simulink model "full_model"  (R2021a)
settings: Solver=FixedStepAuto  StartTime=0.0  StopTime=conf.cycle.stop  FixedStep=conf.time.step  RelTol=1e-3
InitFcn:
  | full_model_init
values from neighbouring files (symbols this model uses):
  bottomCool = abs(conf.cooling.b.x) + abs(conf.cooling.b.y) == 1    [full_model_init.m]
  cellsP = conf.cells.p    [full_model_init.m]
  cellsS = conf.modules.x*conf.modules.y*conf.cells.s    [full_model_init.m]
  elecC1 = C1_matrix*elecCellCap/cellCapGiant    [full_model_init.m]
  elecCellCap = 60    [full_model_init.m]
  elecInitSOC = (1 - variation)*socAve + 2*variation*socAve*rand(cellsS,cellsP)    [full_model_init.m]
  elecLoadDenomInds = 0    [full_model_init.m]
  elecLoadTerm12Inds = 0    [full_model_init.m]
  elecLoadTerm1Inds = 0    [full_model_init.m]
  elecLoadTerm2Inds = 0    [full_model_init.m]
  elecLoadTerm3Inds = 0    [full_model_init.m]
  elecOCV = Em_matrix    [full_model_init.m]
  elecR0 = R1_matrix*cellCapGiant/elecCellCap    [full_model_init.m]
  elecR1 = R2_matrix*cellCapGiant/elecCellCap    [full_model_init.m]
  elecSOCBreak = SOC_breakpoints    [full_model_init.m]
  elecTempBreak = Temp_breakpoints    [full_model_init.m]
  maxFlow = min([maxFlowX maxFlowY])    [full_model_init.m]
  mdotDistX = mdotDistX*flowMult    [full_model_init.m]
  mdotDistY = mdotDistY*flowMult    [full_model_init.m]
  n = n + 1    (= 5)    [plot_lines.m]    (also in plot_volumes.m = 2)
  tempAmb = conf.bound.amb    [full_model_init.m]    (also in order_reduction_script.m = data.tempAmb)
  tempTarget = 25    [full_model_init.m]
  thermBoundXA = conf.bound.amb    [full_model_init.m]
  thermBoundXB = conf.bound.amb    [full_model_init.m]
  thermBoundYA = conf.bound.amb    [full_model_init.m]
  thermBoundYB = conf.bound.amb    [full_model_init.m]
  thermBoundZA = conf.bound.amb    [full_model_init.m]
  thermBoundZB = conf.bound.amb    [full_model_init.m]
  thermCellVols = (thermHeatInds ~= 0)    [full_model_init.m]
  thermCp = matDict.Mass_Cp(thermMatID)    [full_model_init.m]
  thermHeatCellToVol = 1/(conf.regions.l*conf.regions.w*conf.regions.t)    [full_model_init.m]
  thermInitTemp = tempAmb*ones(thermDims)+ conf.bound.initBias    [full_model_init.m]
  thermKx = tempK.x    [full_model_init.m]
  thermKy = tempK.y    [full_model_init.m]
  thermKz = tempK.z    [full_model_init.m]
  thermM = rho.*V    [full_model_init.m]
  thermTempInds = zeros(conf.regions.l*conf.regions.w*conf.regions.t,1,cellsS*cellsP)    [full_model_init.m]
  topCool = abs(conf.cooling.t.x) + abs(conf.cooling.t.y) == 1    [full_model_init.m]
  vehAf = 3.15    [full_model_init.m]
  vehCd = 0.28    [full_model_init.m]
  vehM = 2565    [full_model_init.m]
  vehPowerMult = modelEnergy/packEnergy    [full_model_init.m]
undefined symbols (not defined in the file or in its folder): conf, radAirVelBreakPoints, radCoolFlowBreakPoints, radNomFlowMatrix, refAirVelBreakPoints, refCoolFlowBreakPoints, refCoolInTempBreakPoints, refTempOutMatrix, thermDims
libraries: visionstatistics x1
settings Model: Creator=sjtho  LastModifiedBy=sjtho
settings OptimizationCC: OptimizeBlockIOStorage=off  OptimizeDataStoreBuffers=off  BusAssignmentInplaceUpdate=off
settings DebuggingCC: UniqueDataStoreMsg=error  SFUnexpectedBacktrackingDiag=warning  SFNoUnconditionalDefaultTransitionDiag=warning
settings RTWCC: GenerateReport=on  BuildConfiguration=Debug  LaunchReport=on
settings CodeAppCC: ForceParamTrailComments=on  MATLABSourceComments=on  EnableCustomComments=on
settings GRTTargetCC: CombineSignalStateStructs=on  SupportVariableSizeSignals=on  MultiInstanceErrorCode=Warning

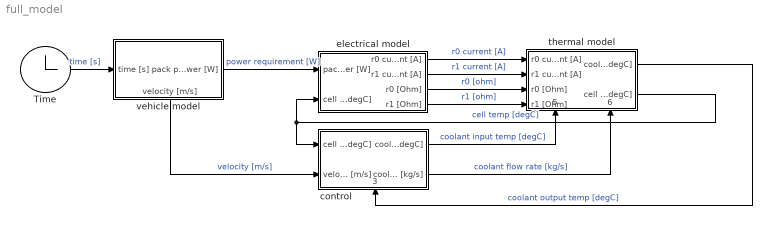
== system full_model ==
  Time : Clock
  control : Subsystem
      settings: PortSchema="{\"entries\":[{\"content\":{\"sides\":[{\"content\":{\"connectorIds\":[\"In1\",\"In2\"]},\"type\":\"ConnectorPlacement.EquallySpacedRectSide\",\"uuid\":\"22f80eaa-bb46-4281-9ec1-3970c1bac2a3\"},{\"content\":{\"connectorIds\":[\"Out1\",\"Out2\"],\"side\":\"RIGHT\"},\"type\":\"ConnectorPlacement.EquallySpacedRectSide\",\"uuid\":\"e76f71c5-d41f-442d-b655-b3bc32395443\"},{\"content\":{\"connectorIds\":[],\"side\":\"TOP\"},\"type\":\"ConnectorPlacement.EquallySpacedRectSide\",\"uuid\":\"e3a9d903-5780-49ee-b4b3-f001d4a3722b\"},{\"content\":{\"connectorIds\":[\"In3\"],\"side\":\"BOTTOM\"},\"type\":\"ConnectorPlacement.EquallySpacedRectSide\",\"uuid\":\"8a36595f-00ae-4362-a59c-271e32328d9e\"}]},\"type\":\"ConnectorPlacement.EquallySpacedConnector\",\"uuid\":\"d37af0d9-ec54-4f0d-b375-47d72f1b804c\"}],\"packageUris\":[\"http://schema.mathworks.com/mf0/Connector/R2020b\"],\"version\":\"1.0\"}"
      mask Display: disp(['Control and ' newline 'Thermal management'])
  electrical model : Subsystem
      mask Display: disp('Electrical Model')
  thermal model : Subsystem
      settings: PortSchema="{\"entries\":[{\"content\":{\"sides\":[{\"content\":{\"connectorIds\":[\"In1\",\"In2\",\"In3\",\"In4\"]},\"type\":\"ConnectorPlacement.EquallySpacedRectSide\",\"uuid\":\"85abd361-fdf9-4e50-9692-c6cfc682c3ac\"},{\"content\":{\"connectorIds\":[\"Out1\",\"Out2\"],\"side\":\"RIGHT\"},\"type\":\"ConnectorPlacement.EquallySpacedRectSide\",\"uuid\":\"50be5dc9-6285-4d3d-a0f1-610cf70c20d6\"},{\"content\":{\"connectorIds\":[],\"side\":\"TOP\"},\"type\":\"ConnectorPlacement.EquallySpacedRectSide\",\"uuid\":\"1bb98c42-8893-43bf-953b-d262aeaa61fe\"},{\"content\":{\"connectorIds\":[\"In5\",\"In6\"],\"side\":\"BOTTOM\"},\"type\":\"ConnectorPlacement.EquallySpacedRectSide\",\"uuid\":\"83d18484-4c30-41fd-9096-006931d5d21f\"}]},\"type\":\"ConnectorPlacement.EquallySpacedConnector\",\"uuid\":\"8afb65a4-2410-4c66-9cd3-3c36ab441c83\"}],\"packageUris\":[\"http://schema.mathworks.com/mf0/Connector/R2020b\"],\"version\":\"1.0\"}"
      mask Display: disp('Thermal Model')
  vehicle model : Subsystem
      settings: PortSchema="{\"entries\":[{\"content\":{\"sides\":[{\"content\":{\"connectorIds\":[\"In1\"]},\"type\":\"ConnectorPlacement.EquallySpacedRectSide\",\"uuid\":\"cf313784-55fc-4068-b83a-27fead484f77\"},{\"content\":{\"connectorIds\":[\"Out1\"],\"side\":\"RIGHT\"},\"type\":\"ConnectorPlacement.EquallySpacedRectSide\",\"uuid\":\"2b8b7e96-e7dc-4089-926d-80148fade29f\"},{\"content\":{\"connectorIds\":[],\"side\":\"TOP\"},\"type\":\"ConnectorPlacement.EquallySpacedRectSide\",\"uuid\":\"332287a3-327f-4bf8-9290-89809e483fea\"},{\"content\":{\"connectorIds\":[\"Out2\"],\"side\":\"BOTTOM\"},\"type\":\"ConnectorPlacement.EquallySpacedRectSide\",\"uuid\":\"f07f6670-fe7e-40c0-9cd8-41a00d5f5993\"}]},\"type\":\"ConnectorPlacement.EquallySpacedConnector\",\"uuid\":\"6bd39f86-8f76-4883-86c4-8a861857bd9f\"}],\"packageUris\":[\"http://schema.mathworks.com/mf0/Connector/R2020b\"],\"version\":\"1.0\"}"
      mask Display: disp('Vehicle Model')
  wires:
  Time/1 -> vehicle model/1(time [s])  "time [s]"
  vehicle model/1(pack power [W]) -> electrical model/1(pack power [W])  "power requirement [W]"
  control/1(coolant input temp [degC]) -> thermal model/5(coolant input temp [degC])  "coolant input temp [degC]"
  control/2(coolant flow rate [kg/s]) -> thermal model/6(coolant flow rate [kg/s])  "coolant flow rate [kg/s]"
  thermal model/1(coolant output temp [degC]) -> control/3(coolant output temp [degC])  "coolant output temp [degC]"
  electrical model/1(r0 current [A]) -> thermal model/1(r0 current [A])  "r0 current [A]"
  electrical model/2(r1 current [A]) -> thermal model/2(r1 current [A])  "r1 current [A]"
  electrical model/3(r0 [Ohm]) -> thermal model/3(r0 [Ohm])  "r0 [ohm]"
  electrical model/4(r1 [Ohm]) -> thermal model/4(r1 [Ohm])  "r1 [ohm]"
  thermal model/2(cell temp [degC]) -> control/1(cell temp [degC]), electrical model/2(cell temp [degC])  "cell temp [degC]"
  vehicle model/2(velocity [m/s]) -> control/2(velocity [m/s])  "velocity [m/s]"

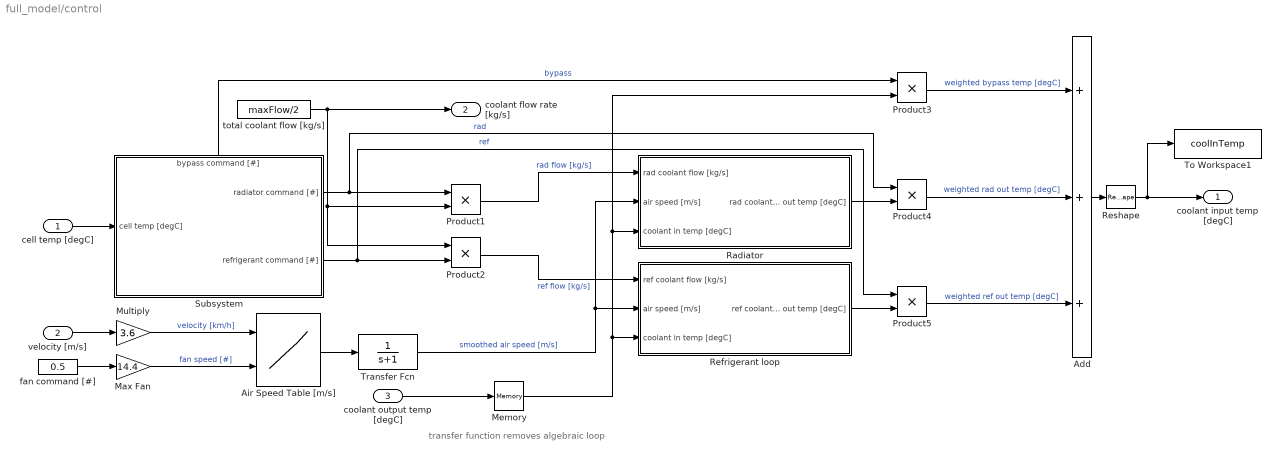
== system full_model/control ==
  note: transfer function removes algebraic loop
  cell temp [degC] : Inport
  velocity [m/s] : Inport  Port=2
  coolant output temp [degC] : Inport  Port=3
  Add : Sum  Inputs=+++
  Air Speed Table [m/s] : Lookup_n-D  BreakpointsForDimension1=[0 40 90 110 150 180 198]  BreakpointsForDimension2=[0 14.4]  IndexSearchMethod=Linear search  BeginIndexSearchUsingPreviousIndexResult=on  Table=[0 0.8 2.2 2.7 3.6 4.1 4.6; 1.5 2.3 3.2 3.5 4.3 4.8 5.1]'  InternalRulePriority=Speed  RndMeth=Simplest  InputSameDT=on
      settings: InputPortMap=u0,u1
  Max Fan : Gain  Gain=14.4
  Memory : Memory  InitialCondition=tempAmb + conf.bound.initBias
  Multiply : Gain  Gain=3.6
  Product{1..5} (5 alike) : Product
  Radiator : Subsystem
  Refrigerant loop : Subsystem
  Reshape : Reshape  OutputDimensionality=Customize  OutputDimensions=1
  Subsystem : Subsystem
      settings: PortSchema="{\"entries\":[{\"content\":{\"sides\":[{\"content\":{\"connectorIds\":[\"In1\"]},\"type\":\"ConnectorPlacement.EquallySpacedRectSide\",\"uuid\":\"39caf9d2-37e9-4ddb-8f89-28cdec2ac0f1\"},{\"content\":{\"connectorIds\":[\"Out1\",\"Out2\"],\"side\":\"RIGHT\"},\"type\":\"ConnectorPlacement.EquallySpacedRectSide\",\"uuid\":\"3cbc02da-b039-4e1d-b42e-efc08ec78021\"},{\"content\":{\"connectorIds\":[\"Out3\"],\"side\":\"TOP\"},\"type\":\"ConnectorPlacement.EquallySpacedRectSide\",\"uuid\":\"b4b3f97e-dd64-49e3-8c52-9947fb1a0732\"}]},\"type\":\"ConnectorPlacement.EquallySpacedConnector\",\"uuid\":\"4860c07b-2c7d-4cd4-976e-5c2ba4e5db64\"}],\"packageUris\":[\"http://schema.mathworks.com/mf0/Connector/R2020b\"],\"version\":\"1.0\"}"
  To Workspace1 : ToWorkspace  VariableName=coolInTemp  SaveFormat=Timeseries  SampleTime=conf.time.sample
  Transfer Fcn : TransferFcn  Denominator=[1 1]
  fan command [#] : Constant  Value=0.5
  total coolant flow [kg/s] : Constant  Value=maxFlow/2
  coolant input temp [degC] : Outport
  coolant flow rate [kg/s] : Outport  Port=2
  wires:
  Max Fan/1 -> Air Speed Table [m/s]/2  "fan speed [#]"
  velocity [m/s]/1 -> Multiply/1
  fan command [#]/1 -> Max Fan/1
  Multiply/1 -> Air Speed Table [m/s]/1  "velocity [km/h]"
  Air Speed Table [m/s]/1 -> Transfer Fcn/1
  cell temp [degC]/1 -> Subsystem/1(cell temp [degC])
  Subsystem/1(radiator command [#]) -> Product1/1, Product4/1  "rad"
  Subsystem/2(refrigerant command [#]) -> Product5/1, Product2/2  "ref"
  Product1/1 -> Radiator/1(rad coolant flow [kg/s])  "rad flow [kg/s]"
  Product2/1 -> Refrigerant loop/1(ref coolant flow [kg/s])  "ref flow [kg/s]"
  Transfer Fcn/1 -> Radiator/2(air speed [m/s]), Refrigerant loop/2(air speed [m/s])  "smoothed air speed [m/s]"
  coolant output temp [degC]/1 -> Memory/1
  Refrigerant loop/1(ref coolant out temp [degC]) -> Product5/2
  Radiator/1(rad coolant out temp [degC]) -> Product4/2
  Product4/1 -> Add/2  "weighted rad out temp [degC]"
  Product5/1 -> Add/3  "weighted ref out temp [degC]"
  Product3/1 -> Add/1  "weighted bypass temp [degC]"
  Subsystem/3(bypass command [#]) -> Product3/1  "bypass"
  total coolant flow [kg/s]/1 -> Product2/1, Product1/2, coolant flow rate [kg/s]/1
  Memory/1 -> Product3/2, Radiator/3(coolant in temp [degC]), Refrigerant loop/3(coolant in temp [degC])
  Add/1 -> Reshape/1
  Reshape/1 -> To Workspace1/1, coolant input temp [degC]/1

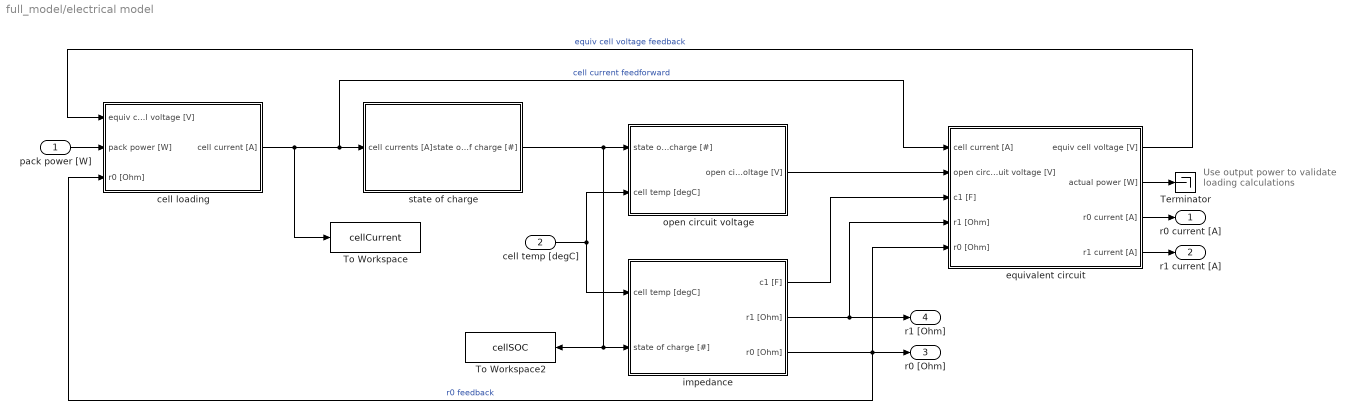
== system full_model/electrical model ==
  note: Use output power to validate loading calculations
  pack power [W] : Inport
  cell temp [degC] : Inport  Port=2
  Terminator : Terminator
  To Workspace : ToWorkspace  VariableName=cellCurrent  SaveFormat=Timeseries  SampleTime=conf.time.sample
  To Workspace2 : ToWorkspace  VariableName=cellSOC  SaveFormat=Timeseries  SampleTime=conf.time.sample
  cell loading : Subsystem
  equivalent circuit : Subsystem
  impedance : Subsystem
  open circuit voltage : Subsystem
  state of charge : Subsystem
  r0 current [A] : Outport
  r1 current [A] : Outport  Port=2
  r0 [Ohm] : Outport  Port=3
  r1 [Ohm] : Outport  Port=4
  wires:
  cell loading/1(cell current [A]) -> To Workspace/1, state of charge/1(cell currents [A]), equivalent circuit/1(cell current [A])  "cell current feedforward"
  cell temp [degC]/1 -> open circuit voltage/2(cell temp [degC]), impedance/1(cell temp [degC])
  state of charge/1(state of charge [#]) -> open circuit voltage/1(state of charge [#]), To Workspace2/1, impedance/2(state of charge [#])
  open circuit voltage/1(open circuit voltage [V]) -> equivalent circuit/2(open circuit voltage [V])
  equivalent circuit/2(actual power [W]) -> Terminator/1
  equivalent circuit/3(r0 current [A]) -> r0 current [A]/1
  equivalent circuit/4(r1 current [A]) -> r1 current [A]/1
  equivalent circuit/1(equiv cell voltage [V]) -> cell loading/1(equiv cell voltage [V])  "equiv cell voltage feedback"
  pack power [W]/1 -> cell loading/2(pack power [W])
  impedance/1(c1 [F]) -> equivalent circuit/3(c1 [F])
  impedance/2(r1 [Ohm]) -> r1 [Ohm]/1, equivalent circuit/4(r1 [Ohm])
  impedance/3(r0 [Ohm]) -> r0 [Ohm]/1, cell loading/3(r0 [Ohm]), equivalent circuit/5(r0 [Ohm])  "r0 feedback"

== system full_model/thermal model ==
  r0 current [A] : Inport
  r1 current [A] : Inport  Port=2
  r0 [Ohm] : Inport  Port=3
  r1 [Ohm] : Inport  Port=4
  coolant input temp [degC] : Inport  Port=5
  coolant flow rate [kg/s] : Inport  Port=6
  Sum1 : Sum  Inputs=|++
  cell temp : Subsystem
      mask Display: disp('Cell Temp')
  coolant flux : Subsystem
      mask Display: disp('Coolant Transfer')
  heat generation : Subsystem
      mask Display: disp('Heat Generation')
  coolant output temp [degC] : Outport
  cell temp [degC] : Outport  Port=2
  wires:
  cell temp/2(volume temp [degC]) -> coolant flux/3(volume temp [K])  "volume temp [degC]"
  coolant input temp [degC]/1 -> coolant flux/1(coolant input temp [K])
  coolant flow rate [kg/s]/1 -> coolant flux/2(coolant flow rate [kg/s])
  r0 current [A]/1 -> heat generation/1(r0 current [A])
  r1 current [A]/1 -> heat generation/2(r1 current [A])
  r0 [Ohm]/1 -> heat generation/3(r0 [Ohm])
  r1 [Ohm]/1 -> heat generation/4(r1 [Ohm])
  heat generation/1(volume heat generation [W]) -> Sum1/1  "volume heat generation [W]"
  cell temp/1(cell temp [degC]) -> cell temp [degC]/1
  Sum1/1 -> cell temp/1(net heat gain [W])  "net heat gain [W]"
  coolant flux/2(coolant output temp [degC]) -> coolant output temp [degC]/1
  coolant flux/1(volume coolant flux [W]) -> Sum1/2

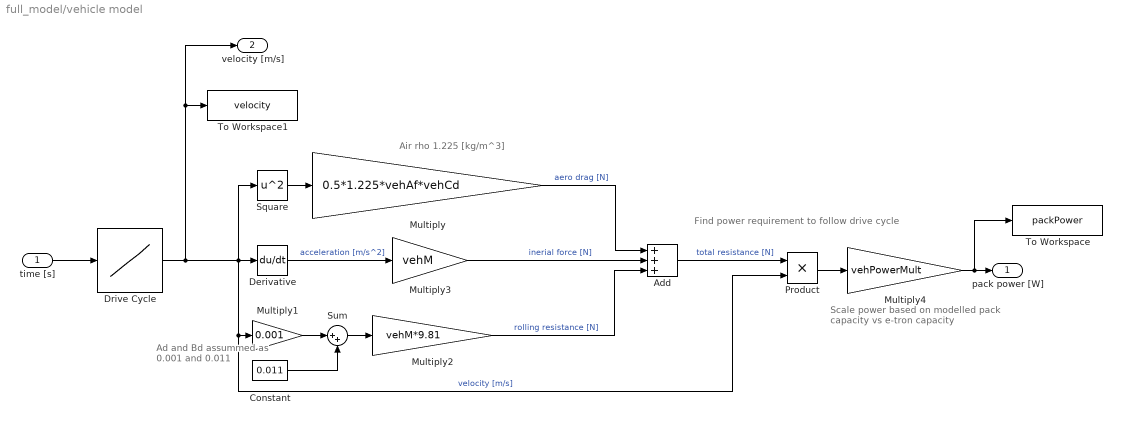
== system full_model/vehicle model ==
  note: Scale power based on modelled pack capacity vs e-tron capacity
  note: Ad and Bd assummed as 0.001 and 0.011
  note: Air rho 1.225 [kg/m^3]
  note: Find power requirement to follow drive cycle
  time [s] : Inport
  Add : Sum  Inputs=+++
  Constant : Constant  Value=0.011
  Derivative : Derivative
  Drive Cycle : Lookup_n-D  NumberOfTableDimensions=1  BreakpointsForDimension1=conf.cycle.time  Table=conf.cycle.vel  InterpMethod=Cubic spline  InternalRulePriority=Speed  RndMeth=Simplest  InputSameDT=on
  Multiply : Gain  Gain=0.5*1.225*vehAf*vehCd
  Multiply1 : Gain  Gain=0.001
  Multiply2 : Gain  Gain=vehM*9.81
  Multiply3 : Gain  Gain=vehM
  Multiply4 : Gain  Gain=vehPowerMult
  Product : Product
  Square : Math  Operator=square  SaturateOnIntegerOverflow=on
  Sum : Sum  Inputs=|++
  To Workspace : ToWorkspace  VariableName=packPower  SaveFormat=Timeseries  SampleTime=conf.time.sample
  To Workspace1 : ToWorkspace  VariableName=velocity  SaveFormat=Timeseries  SampleTime=conf.time.sample
  pack power [W] : Outport
  velocity [m/s] : Outport  Port=2
  wires:
  time [s]/1 -> Drive Cycle/1
  Multiply/1 -> Add/1  "aero drag [N]"
  Drive Cycle/1 -> velocity [m/s]/1, To Workspace1/1, Derivative/1, Multiply1/1, Product/2, Square/1  "velocity [m/s]"
  Add/1 -> Product/1  "total resistance [N]"
  Multiply3/1 -> Add/2  "inerial force [N]"
  Square/1 -> Multiply/1
  Multiply1/1 -> Sum/1
  Derivative/1 -> Multiply3/1  "acceleration [m/s^2]"
  Sum/1 -> Multiply2/1
  Constant/1 -> Sum/2
  Multiply2/1 -> Add/3  "rolling resistance [N]"
  Product/1 -> Multiply4/1
  Multiply4/1 -> To Workspace/1, pack power [W]/1

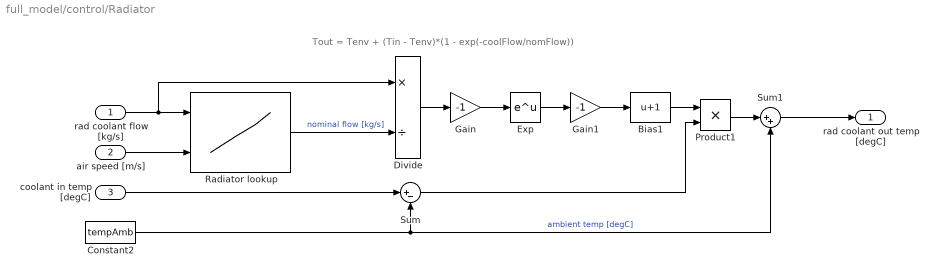
== system full_model/control/Radiator ==
  note: Tout = Tenv + (Tin - Tenv)*(1 - exp(-coolFlow/nomFlow))
  rad coolant flow [kg/s] : Inport
  air speed [m/s] : Inport  Port=2
  coolant in temp [degC] : Inport  Port=3
  Bias1 : Bias  Bias=1
  Constant2 : Constant  Value=tempAmb
  Divide : Product  Inputs=*/
  Exp : Math  SaturateOnIntegerOverflow=on
  Gain : Gain  Gain=-1
  Gain1 : Gain  Gain=-1
  Product1 : Product
  Radiator lookup : Lookup_n-D  BreakpointsForDimension1=radCoolFlowBreakPoints  BreakpointsForDimension2=radAirVelBreakPoints  BreakpointsForDimension3=refCoolInTempBreakPoints  Table=radNomFlowMatrix  InternalRulePriority=Speed  RndMeth=Simplest  InputSameDT=on
      settings: InputPortMap=u0,u1
  Sum : Sum  Inputs=|+-
  Sum1 : Sum  Inputs=|++
  rad coolant out temp [degC] : Outport
  wires:
  Radiator lookup/1 -> Divide/2  "nominal flow [kg/s]"
  Product1/1 -> Sum1/1
  rad coolant flow [kg/s]/1 -> Divide/1, Radiator lookup/1
  air speed [m/s]/1 -> Radiator lookup/2
  Divide/1 -> Gain/1
  Gain/1 -> Exp/1
  Exp/1 -> Gain1/1
  Gain1/1 -> Bias1/1
  Bias1/1 -> Product1/1
  coolant in temp [degC]/1 -> Sum/1
  Constant2/1 -> Sum1/2, Sum/2  "ambient temp [degC]"
  Sum/1 -> Product1/2
  Sum1/1 -> rad coolant out temp [degC]/1

== system full_model/control/Refrigerant loop ==
  ref coolant flow [kg/s] : Inport
  air speed [m/s] : Inport  Port=2
  coolant in temp [degC] : Inport  Port=3
  Refrigerant Loop : Lookup_n-D  NumberOfTableDimensions=3  BreakpointsForDimension1=refCoolFlowBreakPoints  BreakpointsForDimension2=refAirVelBreakPoints  BreakpointsForDimension3=refCoolInTempBreakPoints  Table=refTempOutMatrix  InternalRulePriority=Speed  RndMeth=Simplest  InputSameDT=on
      settings: InputPortMap=u0,u1,u2
  ref coolant out temp [degC] : Outport
  wires:
  air speed [m/s]/1 -> Refrigerant Loop/2
  coolant in temp [degC]/1 -> Refrigerant Loop/3
  Refrigerant Loop/1 -> ref coolant out temp [degC]/1
  ref coolant flow [kg/s]/1 -> Refrigerant Loop/1

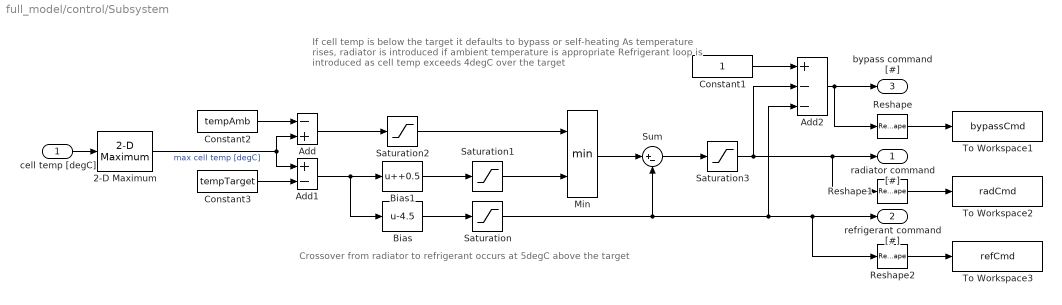
== system full_model/control/Subsystem ==
  note: Crossover from radiator to refrigerant occurs at 5degC above the target
  note: If cell temp is below the target it defaults to bypass or self-heating
      | As temperature rises, radiator is introduced if ambient temperature is appropriate
      | Refrigerant loop is introduced as cell temp exceeds 4degC over the target
  cell temp [degC] : Inport
  2-D Maximum : visionstatistics/2-D Maximum  fcn=Value  reset=None  indexBase=One  operateOver=Entire input  Dimension=1  colComp=on  operation=maximum  accumLastDataTypeStr=Inherit: Same as product output  roiEnable=off  roiType=Rectangles  roiPortion=Entire ROI  roiOutput=Individual statistics for each ROI  roiFlag=off  roundingMode=Floor  overflowMode=off  accumDataTypeStr=Inherit: Same as product output
      settings: SourceProductBaseCode=VP
  Add : Sum  Inputs=-+
  Add1 : Sum  Inputs=+-
  Add2 : Sum  Inputs=+--
  Bias : Bias  Bias=-4.5
  Bias1 : Bias  Bias=+0.5
  Constant1 : Constant
  Constant2 : Constant  Value=tempAmb
  Constant3 : Constant  Value=tempTarget
  Min : MinMax  Inputs=2
  Reshape : Reshape
  Reshape1 : Reshape
  Reshape2 : Reshape
  Saturation{,1..3} (4 alike) : Saturate  UpperLimit=1  LowerLimit=0
  Sum : Sum  Inputs=|+-
  To Workspace1 : ToWorkspace  VariableName=bypassCmd  SaveFormat=Timeseries  SampleTime=conf.time.sample
  To Workspace2 : ToWorkspace  VariableName=radCmd  SaveFormat=Timeseries  SampleTime=conf.time.sample
  To Workspace3 : ToWorkspace  VariableName=refCmd  SaveFormat=Timeseries  SampleTime=conf.time.sample
  radiator command [#] : Outport
  refrigerant command [#] : Outport  Port=2
  bypass command [#] : Outport  Port=3
  wires:
  cell temp [degC]/1 -> 2-D Maximum/1
  2-D Maximum/1 -> Add1/1, Add/2  "max cell temp [degC]"
  Constant3/1 -> Add1/2
  Constant2/1 -> Add/1
  Add1/1 -> Bias1/1, Bias/1
  Bias/1 -> Saturation/1
  Saturation/1 -> Add2/3, Reshape2/1, refrigerant command [#]/1, Sum/2
  Add/1 -> Saturation2/1
  Bias1/1 -> Saturation1/1
  Saturation2/1 -> Min/1
  Saturation1/1 -> Min/2
  Min/1 -> Sum/1
  Sum/1 -> Saturation3/1
  Saturation3/1 -> Reshape1/1, radiator command [#]/1, Add2/2
  Constant1/1 -> Add2/1
  Add2/1 -> Reshape/1, bypass command [#]/1
  Reshape/1 -> To Workspace1/1
  Reshape1/1 -> To Workspace2/1
  Reshape2/1 -> To Workspace3/1

== system full_model/electrical model/cell loading ==
  note: Using if statement to calculate cell current in the correct way. This varies based on the number of parallel cells
  equiv cell voltage [V] : Inport
  pack power [W] : Inport  Port=2
  r0 [Ohm] : Inport  Port=3
  Cell Loading Function : MATLAB Function  TreatAsAtomicUnit=on
  Pack current : Subsystem
  Pack voltage and resistance : Subsystem
  Reshape : Reshape  OutputDimensionality=Customize  OutputDimensions=1
  cell current [A] : Outport
  wires:
  r0 [Ohm]/1 -> Cell Loading Function/3(r0Mat), Pack voltage and resistance/2(r0 [Ohm])
  Pack voltage and resistance/1(pack thevenin voltage [V]) -> Pack current/1(pack thevenin voltage [V])
  Pack voltage and resistance/2(pack thevenin resistance [Ohm]) -> Pack current/2(pack thevenin resistance [Ohm])
  pack power [W]/1 -> Pack current/3(pack power [W])
  equiv cell voltage [V]/1 -> Cell Loading Function/1(veqMat), Pack voltage and resistance/1(equiv cell voltage [V])
  Cell Loading Function/1(cellCurrent) -> cell current [A]/1
  Reshape/1 -> Cell Loading Function/2(ibat)
  Pack current/1(pack current [A]) -> Reshape/1

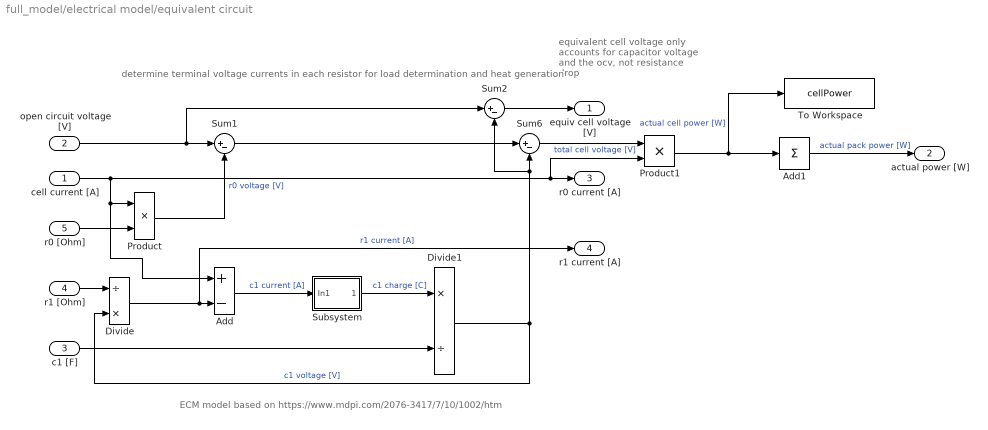
== system full_model/electrical model/equivalent circuit ==
  note: equivalent cell voltage only accounts for capacitor voltage and the ocv, not resistance drop
  note: determine terminal voltage currents in each resistor for load determination and heat generation
  note: ECM model based on https://www.mdpi.com/2076-3417/7/10/1002/htm
  cell current [A] : Inport
  open circuit voltage [V] : Inport  Port=2
  c1 [F] : Inport  Port=3
  r1 [Ohm] : Inport  Port=4
  r0 [Ohm] : Inport  Port=5
  Add : Sum  Inputs=+-
  Add1 : Sum  Inputs=+
  Divide : Product  Inputs=/*
  Divide1 : Product  Inputs=*/
  Product : Product
  Product1 : Product
  Subsystem : Subsystem
      mask Display: disp('DT Int');
  Sum1 : Sum  Inputs=|+-
  Sum2 : Sum  Inputs=|+-
  Sum6 : Sum  Inputs=|+-
  To Workspace : ToWorkspace  VariableName=cellPower  SaveFormat=Timeseries  SampleTime=conf.time.sample
  equiv cell voltage [V] : Outport
  actual power [W] : Outport  Port=2
  r0 current [A] : Outport  Port=3
  r1 current [A] : Outport  Port=4
  wires:
  Add/1 -> Subsystem/1(In1)  "c1 current [A]"
  Subsystem/1(Out1) -> Divide1/1  "c1 charge [C]"
  Divide/1 -> r1 current [A]/1, Add/2  "r1 current [A]"
  Sum1/1 -> Sum6/1
  Product/1 -> Sum1/2  "r0 voltage [V]"
  c1 [F]/1 -> Divide1/2
  Divide1/1 -> Divide/2, Sum2/2, Sum6/2  "c1 voltage [V]"
  open circuit voltage [V]/1 -> Sum2/1, Sum1/1
  cell current [A]/1 -> Product1/2, r0 current [A]/1, Product/1, Add/1
  r0 [Ohm]/1 -> Product/2
  r1 [Ohm]/1 -> Divide/1
  Sum2/1 -> equiv cell voltage [V]/1
  Sum6/1 -> Product1/1  "total cell voltage [V]"
  Product1/1 -> To Workspace/1, Add1/1  "actual cell power [W]"
  Add1/1 -> actual power [W]/1  "actual pack power [W]"

== system full_model/electrical model/impedance ==
  note: Impedence determination using 2D look-up table with state of charge and temperature
  cell temp [degC] : Inport
  state of charge [#] : Inport  Port=2
  Capacitance 1 : Lookup_n-D  BreakpointsForDimension1=elecTempBreak  BreakpointsForDimension2=elecSOCBreak  Table=elecC1  InternalRulePriority=Speed  RndMeth=Simplest  InputSameDT=on
      settings: InputPortMap=u0,u1
  Resistance 0 : Lookup_n-D  BreakpointsForDimension1=elecTempBreak  BreakpointsForDimension2=elecSOCBreak  Table=elecR0  InternalRulePriority=Speed  RndMeth=Simplest  InputSameDT=on
      settings: InputPortMap=u0,u1
  Resistance 1 : Lookup_n-D  BreakpointsForDimension1=elecTempBreak  BreakpointsForDimension2=elecSOCBreak  Table=elecR1  InternalRulePriority=Speed  RndMeth=Simplest  InputSameDT=on
      settings: InputPortMap=u0,u1
  c1 [F] : Outport
  r1 [Ohm] : Outport  Port=2
  r0 [Ohm] : Outport  Port=3
  wires:
  state of charge [#]/1 -> Resistance 0/2, Resistance 1/2, Capacitance 1/2  "SOC [#]"
  Resistance 0/1 -> r0 [Ohm]/1
  Resistance 1/1 -> r1 [Ohm]/1
  Capacitance 1/1 -> c1 [F]/1
  cell temp [degC]/1 -> Capacitance 1/1, Resistance 1/1, Resistance 0/1  "cell temp [degC]"

== system full_model/electrical model/open circuit voltage ==
  note: Open circuit voltage determination using 2D look-up table with state of charge and temperature
  state of charge [#] : Inport
  cell temp [degC] : Inport  Port=2
  Open Circuit Voltage : Lookup_n-D  BreakpointsForDimension1=elecTempBreak  BreakpointsForDimension2=elecSOCBreak  Table=elecOCV  InternalRulePriority=Speed  RndMeth=Simplest  InputSameDT=on
      settings: InputPortMap=u0,u1
  open circuit voltage [V] : Outport
  wires:
  state of charge [#]/1 -> Open Circuit Voltage/2
  Open Circuit Voltage/1 -> open circuit voltage [V]/1
  cell temp [degC]/1 -> Open Circuit Voltage/1

== system full_model/electrical model/state of charge ==
  note: -1 as positive current in the model is discharge
  cell currents [A] : Inport
  Multiply : Gain  Gain=1/3600
  Multiply1 : Gain  Gain=-1/elecCellCap
  Subsystem : Subsystem
      mask Display: disp('DT Int');
  state of charge [#] : Outport
  wires:
  cell currents [A]/1 -> Multiply/1  "current [A]"
  Multiply1/1 -> Subsystem/1(In1)  "discharge normalised [#]"
  Multiply/1 -> Multiply1/1  "current [Hourly]"
  Subsystem/1(Out1) -> state of charge [#]/1  "soc [#]"

== system full_model/thermal model/cell temp ==
  net heat gain [W] : Inport
  Finite Volume Model : Subsystem
  To Workspace : ToWorkspace  VariableName=volTemp  SaveFormat=Timeseries  SampleTime=conf.time.sample
  To Workspace1 : ToWorkspace  VariableName=cellTemp  SaveFormat=Timeseries  SampleTime=conf.time.sample
  map volume temp to cells : MATLAB Function  TreatAsAtomicUnit=on
  cell temp [degC] : Outport
  volume temp [degC] : Outport  Port=2
  wires:
  Finite Volume Model/1(volume temp [degC]) -> To Workspace/1, map volume temp to cells/1(volTemp), volume temp [degC]/1
  net heat gain [W]/1 -> Finite Volume Model/1(net heat gain [W])
  map volume temp to cells/1(cellTemp) -> To Workspace1/1, cell temp [degC]/1

== system full_model/thermal model/coolant flux ==
  note: Only process coolant heat transfer if cooling is in use
  coolant input temp [K] : Inport
  coolant flow rate [kg/s] : Inport  Port=2
  volume temp [K] : Inport  Port=3
  Constant : Constant  Value=topCool
  Constant1 : Constant  Value=bottomCool
  If : If
  If Action Subsystem : Subsystem  TreatAsAtomicUnit=on
  If Action Subsystem1 : Subsystem  TreatAsAtomicUnit=on
  Merge : Merge
  Merge1 : Merge
  Sum2 : Sum  Inputs=|++
  To Workspace1 : ToWorkspace  VariableName=coolOutTemp  SaveFormat=Timeseries  SampleTime=conf.time.sample
  volume coolant flux [W] : Outport
  coolant output temp [degC] : Outport  Port=2
  wires:
  coolant input temp [K]/1 -> If Action Subsystem/1(coolant input temp [degC])
  Constant/1 -> Sum2/1
  Constant1/1 -> Sum2/2
  Sum2/1 -> If/1
  If/1 -> If Action Subsystem/Action
  If/2 -> If Action Subsystem1/Action
  If Action Subsystem/1(volume coolant flux [W]) -> Merge/1
  If Action Subsystem/2(coolant output temp [degC]) -> Merge1/1
  If Action Subsystem1/1(volume coolant flux [W]) -> Merge/2
  If Action Subsystem1/2(coolant output temp [degC]) -> Merge1/2
  coolant flow rate [kg/s]/1 -> If Action Subsystem/2(coolant flow rate [kg/s])
  volume temp [K]/1 -> If Action Subsystem/3(volume temp [degC])
  Merge1/1 -> coolant output temp [degC]/1, To Workspace1/1
  Merge/1 -> volume coolant flux [W]/1

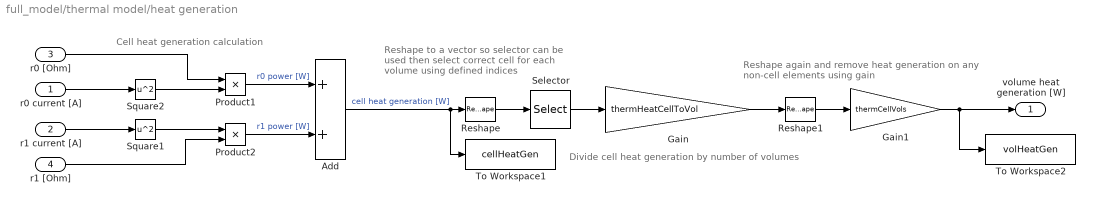
== system full_model/thermal model/heat generation ==
  note: Reshape again and remove heat generation on any non-cell elements using gain
  note: Divide cell heat generation by number of volumes
  note: Reshape to a vector so selector can be used then select correct cell for each volume using defined indices
  note: Cell heat generation calculation
  r0 current [A] : Inport
  r1 current [A] : Inport  Port=2
  r0 [Ohm] : Inport  Port=3
  r1 [Ohm] : Inport  Port=4
  Add : Sum
  Gain : Gain  Gain=thermHeatCellToVol
  Gain1 : Gain  Gain=thermCellVols
  Product1 : Product
  Product2 : Product
  Reshape : Reshape
  Reshape1 : Reshape  OutputDimensionality=Customize  OutputDimensions=thermDims
  Selector : Selector  InputPortWidth=cellsS*cellsP  IndexOptions=Index vector (dialog)  Indices=thermHeatIndsNo0  OutputSizes=1
  Square1 : Math  Operator=square  SaturateOnIntegerOverflow=on
  Square2 : Math  Operator=square  SaturateOnIntegerOverflow=on
  To Workspace1 : ToWorkspace  VariableName=cellHeatGen  SaveFormat=Timeseries  SampleTime=conf.time.sample
  To Workspace2 : ToWorkspace  VariableName=volHeatGen  SaveFormat=Timeseries  SampleTime=conf.time.sample
  volume heat generation [W] : Outport
  wires:
  Square1/1 -> Product2/1
  Product2/1 -> Add/2  "r1 power [W]"
  Square2/1 -> Product1/2
  r0 current [A]/1 -> Square2/1
  r1 current [A]/1 -> Square1/1
  r0 [Ohm]/1 -> Product1/1
  r1 [Ohm]/1 -> Product2/2
  Product1/1 -> Add/1  "r0 power [W]"
  Gain/1 -> Reshape1/1
  Selector/1 -> Gain/1
  Reshape/1 -> Selector/1
  Add/1 -> Reshape/1, To Workspace1/1  "cell heat generation [W]"
  Reshape1/1 -> Gain1/1
  Gain1/1 -> volume heat generation [W]/1, To Workspace2/1

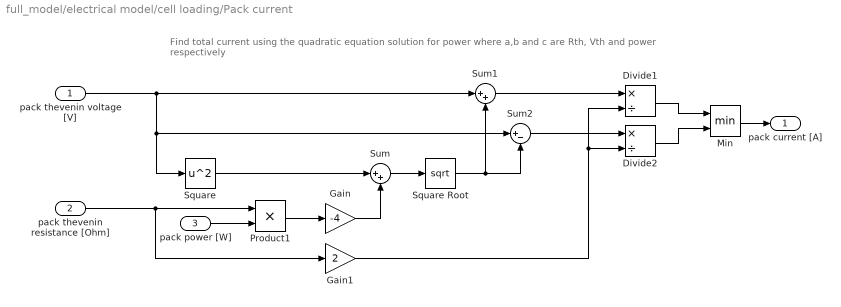
== system full_model/electrical model/cell loading/Pack current ==
  note: Find total current using the quadratic equation solution for power where a,b and c are Rth, Vth and power respectively
  pack thevenin voltage [V] : Inport
  pack thevenin resistance [Ohm] : Inport  Port=2
  pack power [W] : Inport  Port=3
  Divide1 : Product  Inputs=*/
  Divide2 : Product  Inputs=*/
  Gain : Gain  Gain=-4
  Gain1 : Gain  Gain=2
  Min : MinMax  Inputs=2
  Product1 : Product
  Square : Math  Operator=square  SaturateOnIntegerOverflow=on
  Square Root : Sqrt  SaturateOnIntegerOverflow=on
  Sum : Sum  Inputs=|++
  Sum1 : Sum  Inputs=|++
  Sum2 : Sum  Inputs=|+-
  pack current [A] : Outport
  wires:
  pack thevenin voltage [V]/1 -> Square/1, Sum2/1, Sum1/1
  Square/1 -> Sum/1
  Sum/1 -> Square Root/1
  pack thevenin resistance [Ohm]/1 -> Gain1/1, Product1/1
  Gain1/1 -> Divide2/2, Divide1/2
  Divide2/1 -> Min/2
  Square Root/1 -> Sum1/2, Sum2/2
  Sum2/1 -> Divide2/1
  Sum1/1 -> Divide1/1
  Divide1/1 -> Min/1
  Gain/1 -> Sum/2
  Product1/1 -> Gain/1
  pack power [W]/1 -> Product1/2
  Min/1 -> pack current [A]/1

== system full_model/electrical model/cell loading/Pack voltage and resistance ==
  note: Find pack voltage and resistance for the pack using a combination of norton and thevenin equivalent circuits
  equiv cell voltage [V] : Inport
  r0 [Ohm] : Inport  Port=2
  Divide : Product  Inputs=*/
  Math Function1 : Math  Operator=reciprocal  SaturateOnIntegerOverflow=on
  Math Function2 : Math  Operator=reciprocal  SaturateOnIntegerOverflow=on
  Product : Product
  Sum of Elements : Sum  Inputs=+  CollapseMode=Specified dimension  CollapseDim=2
  Sum of Elements1 : Sum  Inputs=+  CollapseMode=Specified dimension  CollapseDim=2
  Sum of Elements2 : Sum  Inputs=+  CollapseMode=Specified dimension
  Sum of Elements3 : Sum  Inputs=+  CollapseMode=Specified dimension
  pack thevenin voltage [V] : Outport
  pack thevenin resistance [Ohm] : Outport  Port=2
  wires:
  Sum of Elements1/1 -> Math Function2/1  "parallel inversed r0 [1/Ohm]"
  r0 [Ohm]/1 -> Divide/2, Math Function1/1
  Divide/1 -> Sum of Elements/1  "cell norton current [A]"
  Sum of Elements/1 -> Product/1  "parallel norton current [A]"
  Math Function2/1 -> Product/2, Sum of Elements3/1  "parallel norton r0 [Ohm]"
  Product/1 -> Sum of Elements2/1  "parallel thevenin voltage [V]"
  Math Function1/1 -> Sum of Elements1/1  "inversed r0 [1/Ohm]"
  Sum of Elements3/1 -> pack thevenin resistance [Ohm]/1
  Sum of Elements2/1 -> pack thevenin voltage [V]/1
  equiv cell voltage [V]/1 -> Divide/1

== system full_model/electrical model/equivalent circuit/Subsystem ==
  note: Discrete time integrator using the time step
  In1 : Inport
  Memory : Memory
  Sum3 : Sum  Inputs=|++
  Time step : Gain  Gain=conf.time.step
  Out1 : Outport
  wires:
  In1/1 -> Time step/1
  Memory/1 -> Out1/1, Sum3/2  "T"
  Sum3/1 -> Memory/1
  Time step/1 -> Sum3/1

== system full_model/electrical model/state of charge/Subsystem ==
  note: Discrete time integrator using the time step
  In1 : Inport
  Memory : Memory  InitialCondition=elecInitSOC
  Sum3 : Sum  Inputs=|++
  Time step : Gain  Gain=conf.time.step
  Out1 : Outport
  wires:
  In1/1 -> Time step/1
  Memory/1 -> Out1/1, Sum3/2  "T"
  Sum3/1 -> Memory/1
  Time step/1 -> Sum3/1

== system full_model/thermal model/cell temp/Finite Volume Model ==
  note: Integrate temp change with a discrete time integrator
  note: Divide temperature differences by thermal resistance for heat flux at boundaries
  note: Combine heat flow into volumes with net heat gain and scale into a temperature change using material properties
  net heat gain [W] : Inport
  Constant2 : Constant  Value=thermKx
  Constant3 : Constant  Value=thermKy
  Constant4 : Constant  Value=thermKz
  Differential 1 : Subsystem
  Differential 2 : Subsystem
  Gain : Gain  Gain=1/thermCp
  Gain1 : Gain  Gain=1/thermM
  Product : Product
  Product1 : Product
  Product2 : Product
  Subsystem : Subsystem
      mask Display: disp('DT Int');
  Sum : Sum  Inputs=|-+
  volume temp [degC] : Outport
  wires:
  Subsystem/1(Out1) -> volume temp [degC]/1, Differential 1/1(volume temp [degC])
  Differential 1/1(temp dif x [degC]) -> Product/1
  Differential 1/2(temp dif y [degC]) -> Product1/1
  Differential 1/3(temp dif z [degC]) -> Product2/1
  Constant3/1 -> Product1/2
  Constant4/1 -> Product2/2
  Product/1 -> Differential 2/1(heat flux x [W])  "heat flux x"
  Product1/1 -> Differential 2/2(heat flux y [W])  "heat flux y"
  Product2/1 -> Differential 2/3(heat flux z [W])  "heat flux z"
  Differential 2/1(volume heat flux [W]) -> Sum/1
  Sum/1 -> Gain/1
  Gain/1 -> Gain1/1
  Gain1/1 -> Subsystem/1(In1)
  Constant2/1 -> Product/2
  net heat gain [W]/1 -> Sum/2

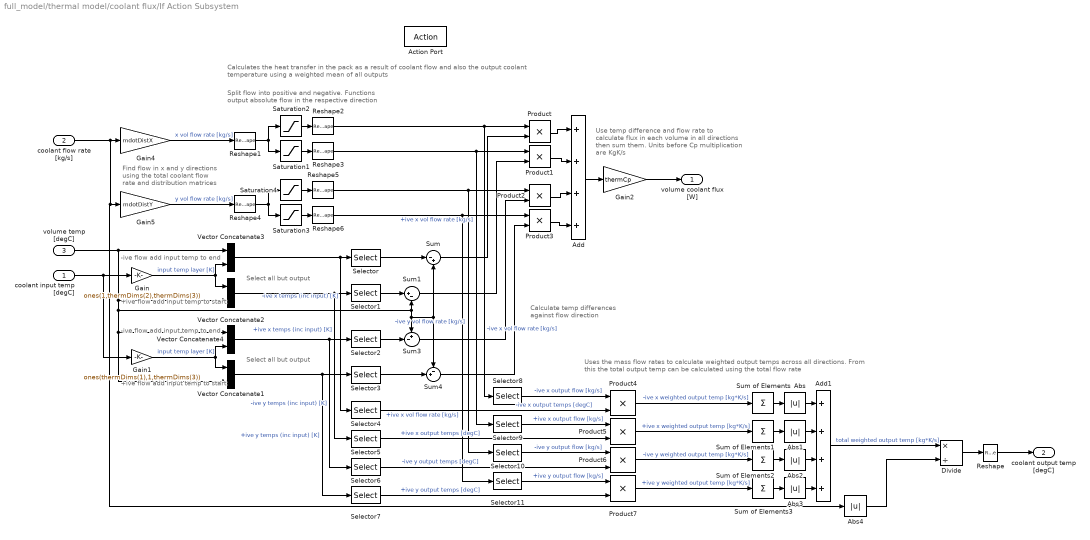
== system full_model/thermal model/coolant flux/If Action Subsystem ==
  note: Find flow in x and y directions using the total coolant flow rate and distribution matrices
  note: Use temp difference and flow rate to calculate flux in each volume in all directions then sum them.
      | Units before Cp multiplication are KgK/s
  note: Calculate temp differences against flow direction
  note: Calculates the heat transfer in the pack as a result of coolant flow and also the output coolant temperature using a weighted mean of all outputs
  note: +ive flow add input temp to start
  note: Uses the mass flow rates to calculate weighted output temps across all directions. From this the total output temp can be calculated using the total flow rate
  note: Select all but output
  note: +ive flow add input temp to start
  note: -ive flow add input temp to end
  note: Split flow into positive and negative. Functions output absolute flow in the respective direction
  note: Select all but output
  note: -ive flow add input temp to end
  coolant input temp [degC] : Inport
  coolant flow rate [kg/s] : Inport  Port=2
  volume temp [degC] : Inport  Port=3
  Action Port : ActionPort  ActionPortLabel=if(u1 > 0)
  Abs{,1..4} (5 alike) : Abs
  Add : Sum  Inputs=++++
  Add1 : Sum  Inputs=++++
  Divide : Product  Inputs=*/
  Gain : Gain  Gain=ones(1,thermDims(2),thermDims(3))
  Gain1 : Gain  Gain=ones(thermDims(1),1,thermDims(3))
  Gain2 : Gain  Gain=thermCp
  Gain4 : Gain  Gain=mdotDistX
  Gain5 : Gain  Gain=mdotDistY
  Product{,1..7} (8 alike) : Product
  Reshape : Reshape  OutputDimensionality=Customize  OutputDimensions=1
  Reshape1 : Reshape  OutputDimensionality=Customize  OutputDimensions=thermDims(1)*thermDims(2)*thermDims(3)
  Reshape{2..3,5..6} (4 alike) : Reshape  OutputDimensionality=Customize  OutputDimensions=thermDims
  Reshape4 : Reshape  OutputDimensionality=Customize  OutputDimensions=thermDims(1)*thermDims(2)*thermDims(3)
  Saturation1 : Saturate  UpperLimit=inf  LowerLimit=0
  Saturation2 : Saturate  UpperLimit=0  LowerLimit=-inf
  Saturation3 : Saturate  UpperLimit=inf  LowerLimit=0
  Saturation4 : Saturate  UpperLimit=0  LowerLimit=-inf
  Selector : Selector  NumberOfDimensions=3  InputPortWidth=3  IndexOptions=Index vector (dialog),Select all,Select all  Indices=2:thermDims(1)+1,1:thermDims(2),1:thermDims(3)  OutputSizes=1,1,1
  Selector1 : Selector  NumberOfDimensions=3  InputPortWidth=3  IndexOptions=Index vector (dialog),Select all,Select all  Indices=1:thermDims(1),1:thermDims(2),1:thermDims(3)  OutputSizes=1,1,1
  Selector10 : Selector  NumberOfDimensions=3  InputPortWidth=3  IndexOptions=Select all,Index vector (dialog),Select all  Indices=1,1,1:thermDims(3)  OutputSizes=1,1,1
  Selector11 : Selector  NumberOfDimensions=3  InputPortWidth=3  IndexOptions=Select all,Index vector (dialog),Select all  Indices=thermDims(1) + 1,thermDims(2),1:thermDims(3)  OutputSizes=1,1,1
  Selector2 : Selector  NumberOfDimensions=3  InputPortWidth=3  IndexOptions=Select all,Index vector (dialog),Select all  Indices=1:thermDims(1),2:thermDims(2)+1,1:thermDims(3)  OutputSizes=1,1,1
  Selector3 : Selector  NumberOfDimensions=3  InputPortWidth=3  IndexOptions=Select all,Index vector (dialog),Select all  Indices=1:thermDims(1),1:thermDims(2),1:thermDims(3)  OutputSizes=1,1,1
  Selector4 : Selector  NumberOfDimensions=3  InputPortWidth=3  IndexOptions=Index vector (dialog),Select all,Select all  Indices=1,1:thermDims(2),1:thermDims(3)  OutputSizes=1,1,1
  Selector5 : Selector  NumberOfDimensions=3  InputPortWidth=3  IndexOptions=Index vector (dialog),Select all,Select all  Indices=thermDims(1) + 1,1:thermDims(2),1:thermDims(3)  OutputSizes=1,1,1
  Selector6 : Selector  NumberOfDimensions=3  InputPortWidth=3  IndexOptions=Select all,Index vector (dialog),Select all  Indices=1,1,1:thermDims(3)  OutputSizes=1,1,1
  Selector7 : Selector  NumberOfDimensions=3  InputPortWidth=3  IndexOptions=Select all,Index vector (dialog),Select all  Indices=thermDims(1) + 1,thermDims(2)+1,1:thermDims(3)  OutputSizes=1,1,1
  Selector8 : Selector  NumberOfDimensions=3  InputPortWidth=3  IndexOptions=Index vector (dialog),Select all,Select all  Indices=1,1:thermDims(2),1:thermDims(3)  OutputSizes=1,1,1
  Selector9 : Selector  NumberOfDimensions=3  InputPortWidth=3  IndexOptions=Index vector (dialog),Select all,Select all  Indices=thermDims(1),1:thermDims(2),1:thermDims(3)  OutputSizes=1,1,1
  Sum : Sum  Inputs=|-+
  Sum of Elements{,1..3} (4 alike) : Sum  Inputs=+
  Sum1 : Sum  Inputs=|+-
  Sum3 : Sum  Inputs=+-|
  Sum4 : Sum  Inputs=-+|
  Vector Concatenate1 : Concatenate  Mode=Multidimensional array  ConcatenateDimension=2
  Vector Concatenate2 : Concatenate  Mode=Multidimensional array
  Vector Concatenate3 : Concatenate  Mode=Multidimensional array
  Vector Concatenate4 : Concatenate  Mode=Multidimensional array  ConcatenateDimension=2
  volume coolant flux [W] : Outport
  coolant output temp [degC] : Outport  Port=2
  wires:
  Gain5/1 -> Reshape4/1  "y vol flow rate [kg/s]"
  Divide/1 -> Reshape/1
  Product7/1 -> Sum of Elements3/1  "+ive y weighted output temp [kg*K/s]"
  Selector10/1 -> Product6/1  "-ive y output flow [kg/s]"
  Product6/1 -> Sum of Elements2/1  "-ive y weighted output temp [kg*K/s]"
  Product5/1 -> Sum of Elements1/1  "+ive x weighted output temp [kg*K/s]"
  Product4/1 -> Sum of Elements/1  "-ive x weighted output temp [kg*K/s]"
  Product3/1 -> Add/4
  Gain2/1 -> volume coolant flux [W]/1
  Selector6/1 -> Product6/2  "-ive y output temps [degC]"
  Selector4/1 -> Product4/2  "-ive x output temps [degC]"
  Reshape6/1 -> Product3/1, Selector11/1  "+ive x vol flow rate [kg/s]"
  Selector9/1 -> Product5/1  "+ive x output flow [kg/s]"
  coolant flow rate [kg/s]/1 -> Abs4/1, Gain5/1, Gain4/1
  Product2/1 -> Add/3
  Product1/1 -> Add/2
  Sum1/1 -> Product1/2
  Selector2/1 -> Sum3/2
  volume temp [degC]/1 -> Vector Concatenate4/1, Vector Concatenate1/2, Sum3/1, Sum4/1, Sum/2, Sum1/2, Vector Concatenate2/2, Vector Concatenate3/1
  Sum/1 -> Product/2
  Gain1/1 -> Vector Concatenate4/2, Vector Concatenate1/1  "input temp layer [K]"
  Vector Concatenate1/1 -> Selector7/1, Selector3/1  "+ive y temps (inc input) [K]"
  Vector Concatenate2/1 -> Selector5/1, Selector1/1  "+ive x temps (inc input) [K]"
  Product/1 -> Add/1
  Reshape2/1 -> Product/1, Selector8/1  "-ive x vol flow rate [kg/s]"
  Selector5/1 -> Product5/2  "+ive x output temps [degC]"
  Selector11/1 -> Product7/1  "+ive y output flow [kg/s]"
  Abs/1 -> Add1/1
  Sum of Elements1/1 -> Abs1/1
  Reshape/1 -> coolant output temp [degC]/1
  Sum of Elements/1 -> Abs/1
  Selector/1 -> Sum/1
  Selector1/1 -> Sum1/1
  Abs4/1 -> Divide/2
  Vector Concatenate4/1 -> Selector6/1, Selector2/1  "-ive y temps (inc input) [K]"
  Selector8/1 -> Product4/1  "-ive x output flow [kg/s]"
  Sum of Elements3/1 -> Abs3/1
  Sum3/1 -> Product2/2
  Add1/1 -> Divide/1  "total weighted output temp [kg*K/s]"
  Abs3/1 -> Add1/4
  Selector3/1 -> Sum4/2
  coolant input temp [degC]/1 -> Gain/1, Gain1/1
  Gain/1 -> Vector Concatenate2/1, Vector Concatenate3/2  "input temp layer [K]"
  Sum4/1 -> Product3/2
  Gain4/1 -> Reshape1/1  "x vol flow rate [kg/s]"
  Reshape3/1 -> Product1/1, Selector9/1  "+ive x vol flow rate [kg/s]"
  Abs2/1 -> Add1/3
  Reshape5/1 -> Product2/1, Selector10/1  "-ive y vol flow rate [kg/s]"
  Vector Concatenate3/1 -> Selector4/1, Selector/1  "-ive x temps (inc input) [K]"
  Sum of Elements2/1 -> Abs2/1
  Abs1/1 -> Add1/2
  Add/1 -> Gain2/1
  Selector7/1 -> Product7/2  "+ive y output temps [degC]"
  Saturation3/1 -> Reshape6/1
  Saturation2/1 -> Reshape2/1
  Saturation4/1 -> Reshape5/1
  Reshape1/1 -> Saturation1/1, Saturation2/1
  Reshape4/1 -> Saturation4/1, Saturation3/1
  Saturation1/1 -> Reshape3/1

== system full_model/thermal model/coolant flux/If Action Subsystem1 ==
  Action Port : ActionPort  ActionPortLabel=else
  Constant : Constant  Value=zeros(thermDims)
  Constant1 : Constant  Value=0
  volume coolant flux [W] : Outport
  coolant output temp [degC] : Outport  Port=2
  wires:
  Constant/1 -> volume coolant flux [W]/1
  Constant1/1 -> coolant output temp [degC]/1

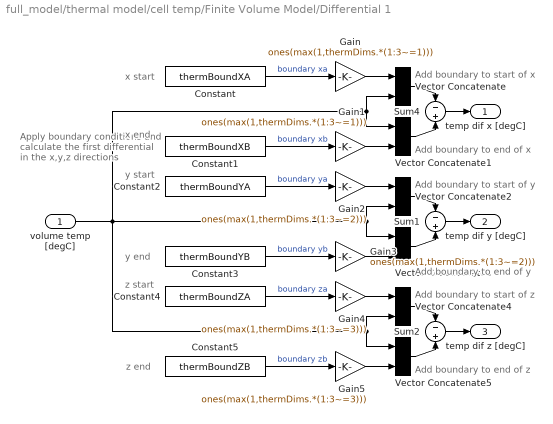
== system full_model/thermal model/cell temp/Finite Volume Model/Differential 1 ==
  note: Add boundary to start of x
  note: Apply boundary conditions and calculate the first differential in the x,y,z directions
  note: z start
  note: y end
  note: x start
  note: x end
  note: y start
  note: z end
  note: Add boundary to end of x
  note: Add boundary to start of y
  note: Add boundary to end of y
  note: Add boundary to start of z
  note: Add boundary to end of z
  volume temp [degC] : Inport
  Constant : Constant  Value=thermBoundXA
  Constant1 : Constant  Value=thermBoundXB
  Constant2 : Constant  Value=thermBoundYA
  Constant3 : Constant  Value=thermBoundYB
  Constant4 : Constant  Value=thermBoundZA
  Constant5 : Constant  Value=thermBoundZB
  Gain : Gain  Gain=ones(max(1,thermDims.*(1:3~=1)))
  Gain1 : Gain  Gain=ones(max(1,thermDims.*(1:3~=1)))
  Gain2 : Gain  Gain=ones(max(1,thermDims.*(1:3~=2)))
  Gain3 : Gain  Gain=ones(max(1,thermDims.*(1:3~=2)))
  Gain4 : Gain  Gain=ones(max(1,thermDims.*(1:3~=3)))
  Gain5 : Gain  Gain=ones(max(1,thermDims.*(1:3~=3)))
  Sum1 : Sum  Inputs=-+
  Sum2 : Sum  Inputs=-+
  Sum4 : Sum  Inputs=-+
  Vector Concatenate : Concatenate  Mode=Multidimensional array
  Vector Concatenate1 : Concatenate  Mode=Multidimensional array
  Vector Concatenate2 : Concatenate  Mode=Multidimensional array  ConcatenateDimension=2
  Vector Concatenate3 : Concatenate  Mode=Multidimensional array  ConcatenateDimension=2
  Vector Concatenate4 : Concatenate  Mode=Multidimensional array  ConcatenateDimension=3
  Vector Concatenate5 : Concatenate  Mode=Multidimensional array  ConcatenateDimension=3
  temp dif x [degC] : Outport
  temp dif y [degC] : Outport  Port=2
  temp dif z [degC] : Outport  Port=3
  wires:
  Vector Concatenate1/1 -> Sum4/2
  Vector Concatenate/1 -> Sum4/1
  Gain/1 -> Vector Concatenate/1
  Gain1/1 -> Vector Concatenate1/2
  Gain3/1 -> Vector Concatenate3/2
  Gain2/1 -> Vector Concatenate2/1
  Vector Concatenate2/1 -> Sum1/1
  Vector Concatenate3/1 -> Sum1/2
  Vector Concatenate5/1 -> Sum2/2
  Vector Concatenate4/1 -> Sum2/1
  Gain4/1 -> Vector Concatenate4/1
  Gain5/1 -> Vector Concatenate5/2
  volume temp [degC]/1 -> Vector Concatenate1/1, Vector Concatenate/2, Vector Concatenate4/2, Vector Concatenate5/1, Vector Concatenate2/2, Vector Concatenate3/1
  Sum4/1 -> temp dif x [degC]/1
  Sum1/1 -> temp dif y [degC]/1
  Sum2/1 -> temp dif z [degC]/1
  Constant2/1 -> Gain2/1  "boundary ya"
  Constant1/1 -> Gain1/1  "boundary xb"
  Constant5/1 -> Gain5/1  "boundary zb"
  Constant4/1 -> Gain4/1  "boundary za"
  Constant3/1 -> Gain3/1  "boundary yb"
  Constant/1 -> Gain/1  "boundary xa"

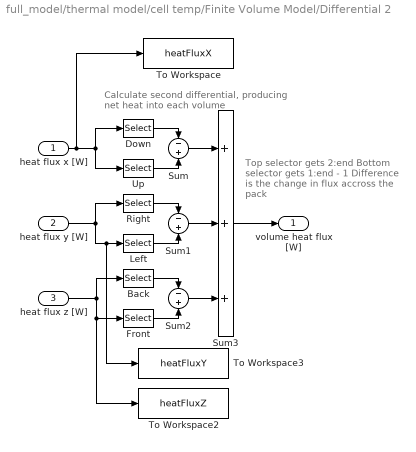
== system full_model/thermal model/cell temp/Finite Volume Model/Differential 2 ==
  note: Top selector gets 2:end
      | Bottom selector gets 1:end - 1
      | Difference is the change in flux
      | accross the pack
  note: Calculate second differential, producing net heat into each volume
  heat flux x [W] : Inport
  heat flux y [W] : Inport  Port=2
  heat flux z [W] : Inport  Port=3
  Back : Selector  NumberOfDimensions=3  IndexMode=Zero-based  InputPortWidth=3  IndexOptions=Select all,Select all,Index vector (dialog)  Indices=[1 1:(n-1)],[2:n n],1:thermDims(3)  OutputSizes=1,1,1
  Down : Selector  NumberOfDimensions=3  IndexMode=Zero-based  InputPortWidth=3  IndexOptions=Index vector (dialog),Select all,Select all  Indices=1:thermDims(1),1,1  OutputSizes=1,1,1
  Front : Selector  NumberOfDimensions=3  InputPortWidth=3  IndexOptions=Select all,Select all,Index vector (dialog)  Indices=[1 1:(n-1)],[1 1:(n-1)],1:thermDims(3)  OutputSizes=1,1,1
  Left : Selector  NumberOfDimensions=3  InputPortWidth=3  IndexOptions=Select all,Index vector (dialog),Select all  Indices=[1 1:(n-1)],1:thermDims(2),1  OutputSizes=1,1,1
  Right : Selector  NumberOfDimensions=3  IndexMode=Zero-based  InputPortWidth=3  IndexOptions=Select all,Index vector (dialog),Select all  Indices=[1 1:(n-1)],1:thermDims(2),1  OutputSizes=1,1,1
  Sum : Sum  Inputs=-+
  Sum1 : Sum  Inputs=-+
  Sum2 : Sum  Inputs=-+
  Sum3 : Sum  Inputs=+++
  To Workspace : ToWorkspace  VariableName=heatFluxX  SaveFormat=Timeseries  SampleTime=conf.time.sample
  To Workspace2 : ToWorkspace  VariableName=heatFluxZ  SaveFormat=Timeseries  SampleTime=conf.time.sample
  To Workspace3 : ToWorkspace  VariableName=heatFluxY  SaveFormat=Timeseries  SampleTime=conf.time.sample
  Up : Selector  NumberOfDimensions=3  InputPortWidth=3  IndexOptions=Index vector (dialog),Select all,Select all  Indices=1:thermDims(1),1,1  OutputSizes=1,1,1
  volume heat flux [W] : Outport
  wires:
  Sum3/1 -> volume heat flux [W]/1
  Back/1 -> Sum2/1
  Front/1 -> Sum2/2
  Down/1 -> Sum/1
  Sum/1 -> Sum3/1
  Up/1 -> Sum/2
  Right/1 -> Sum1/1
  Left/1 -> Sum1/2
  Sum1/1 -> Sum3/2
  Sum2/1 -> Sum3/3
  heat flux y [W]/1 -> To Workspace3/1, Left/1, Right/1
  heat flux z [W]/1 -> Back/1, To Workspace2/1, Front/1
  heat flux x [W]/1 -> To Workspace/1, Up/1, Down/1

== system full_model/thermal model/cell temp/Finite Volume Model/Subsystem ==
  note: Discrete time integrator using the time step
  In1 : Inport
  Memory : Memory  InitialCondition=thermInitTemp
  Sum3 : Sum  Inputs=|++
  Time step : Gain  Gain=conf.time.step
  Out1 : Outport
  wires:
  In1/1 -> Time step/1
  Memory/1 -> Out1/1, Sum3/2  "T"
  Sum3/1 -> Memory/1
  Time step/1 -> Sum3/1

== matlab function full_model/electrical model/cell loading/Cell Loading Function ==
  data: veqMat input; cellCurrent output size=cellsS,cellsP; ibat input; r0Mat input; cellsS parameter; cellsP parameter; elecLoadDenomInds parameter; elecLoadTerm12Inds parameter; elecLoadTerm1Inds parameter; elecLoadTerm2Inds parameter; elecLoadTerm3Inds parameter
function cellCurrent  = cell_loading(veqMat, ibat, r0Mat, cellsS, cellsP, elecLoadDenomInds, elecLoadTerm12Inds, elecLoadTerm1Inds, elecLoadTerm2Inds, elecLoadTerm3Inds)
% Calculate current in each cell
if cellsP == 1
    % All cells take the same current if only in parallel
    term1 = ibat*ones(size(veqMat));   
    term2 = 0; term3 = 0; denom = 1;
elseif cellsP == 2
    % Calculate the current in each cell using pre defined index matrices
    denom = reshape(sum(r0Mat(elecLoadDenomInds)),cellsS,cellsP);
    term1 = veqMat;
    term2 = -reshape(veqMat(elecLoadTerm12Inds),cellsS,cellsP);
    term3 = ibat*reshape(r0Mat(elecLoadTerm12Inds),cellsS,cellsP);
else   
    % Calculate the current in each cell using pre defined index matrices
    denom = reshape(sum(prod(r0Mat(elecLoadDenomInds),2)),cellsS,cellsP);
    term1 = veqMat.*reshape(sum(prod(r0Mat(elecLoadTerm1Inds),2)),cellsS,cellsP);
    term2 = -reshape(sum(veqMat(elecLoadTerm2Inds(:,1,:)).*prod(r0Mat(elecLoadTerm2Inds(:,2:end,:)),2)),cellsS,cellsP);
    term3 = ibat*reshape(prod(r0Mat(elecLoadTerm3Inds)),cellsS,cellsP);
end
cellCurrent = (term1 + term2 + term3)./denom;

== matlab function full_model/thermal model/cell temp/map volume temp to cells ==
  data: volTemp input size=thermDims; cellTemp output size=cellsS,cellsP; thermTempInds parameter; cellsS parameter; cellsP parameter
function cellTemp = fcn(volTemp, thermTempInds, cellsS, cellsP)
% Map volume temperatures to cell format for use in electrical model
cellTemp = reshape(mean(volTemp(thermTempInds),1),cellsS,cellsP);
